simulink model "nncontroller_4_50"  (R2021a)
settings: Solver=VariableStepAuto  StartTime=0.0  StopTime=10.0  RelTol=1e-3
libraries: neural x206
(part 11 of 11)

== system nncontroller_4_50/Feed-Forward Neural Network/Layer 5/Delays 1 ==
  "p{5}" : Inport  PortDimensions=50
      mask Display: e = 0.06;c1 = [120 230 180]/255;c2 = ([120 230 180]+0)/(256+128);c3 = ([120 230 180]+128)/(256+128);patch([0 1 1 0],[0 0 1 1],c1);patch([0 1 1 1-e 1-e 0+e],[0 0 1 1-e 0+e 0+e],c2);patch([0 0 1 1-e 0+e 0+e],[0 1 1 1-e 1-e 0+e],c3);plot([0 1 1 0 0],[0 0 1 1 0]);
  mux : Mux  Inputs=1
      mask Display: e = 0.06;c1 = [120 150 230]/255;c2 = ([120 150 230]+0)/383;c3 = ([120 150 230]+128)/383;patch([0 1 1 0],[0 0 1 1],c1);patch([0 1 1 1-e 1-e 0+e],[0 0 1 1-e 0+e 0+e],c2);patch([0 0 1 1-e 0+e 0+e],[0 1 1 1-e 1-e 0+e],c3);plot([0 1 1 0 0],[0 0 1 1 0]);disp('Mux')
  "pd{5,4}" : Outport
      mask Display: e = 0.06;c1 = [120 230 180]/255;c2 = ([120 230 180]+0)/(256+128);c3 = ([120 230 180]+128)/(256+128);patch([0 1 1 0],[0 0 1 1],c1);patch([0 1 1 1-e 1-e 0+e],[0 0 1 1-e 0+e 0+e],c2);patch([0 0 1 1-e 0+e 0+e],[0 1 1 1-e 1-e 0+e],c3);plot([0 1 1 0 0],[0 0 1 1 0]);
  wires:
  "p{5}"/1 -> mux/1
  mux/1 -> "pd{5,4}"/1

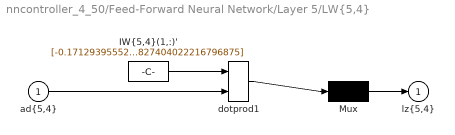
== system nncontroller_4_50/Feed-Forward Neural Network/Layer 5/LW{5,4} ==
  "ad{5,4}" : Inport  PortDimensions=50
      mask Display: e = 0.06;c1 = [120 230 180]/255;c2 = ([120 230 180]+0)/(256+128);c3 = ([120 230 180]+128)/(256+128);patch([0 1 1 0],[0 0 1 1],c1);patch([0 1 1 1-e 1-e 0+e],[0 0 1 1-e 0+e 0+e],c2);patch([0 0 1 1-e 0+e 0+e],[0 1 1 1-e 1-e 0+e],c3);plot([0 1 1 0 0],[0 0 1 1 0]);
  "IW{5,4}(1,:)'" : Constant  Value=[-0.1712939555266810298661539491149596869945526123046875;-0.72795551344690689887784174061380326747894287109375;0.406597786086664469973328550622682087123394012451171875;-0.86752023690311264036978400326916016638278961181640625;0.291551184054806622469868671032600104808807373046875;-0.7823842035386003868069337841006927192211151123046875;-0.9459670471661578705635520236683078110218048095703125;-0.301887099511520984318480032015941105782985687255859375;-0.362312844090777519401314066271879710257053375244140625;0.5028199275581730631756727234460413455963134765625;-0.87837751962319521314981329851434566080570220947265625;-0.289926976234542388421999703496112488210201263427734375;-0.7762515105937903836519353717449121177196502685546875;0.59758198869694301169630534786847420036792755126953125;0.6094541268886020102257816688506864011287689208984375;0.99514085054177059408431205156375654041767120361328125;-0.72455451572289220063538550675730220973491668701171875;-0.37830375588080566995330400459351949393749237060546875;-0.2354275486435387920725048616077401675283908843994140625;1.0042205230011191918748636453528888523578643798828125;0.69321866747018134891078489090432412922382354736328125;0.46433784951853152023204529541544616222381591796875;0.93726104060380410754049762545037083327770233154296875;0.252906313474891952797207750336383469402790069580078125;0.39013454713458373124268518949975259602069854736328125;0.76080914399647803225690267936442978680133819580078125;0.46840297437907174593618719882215373218059539794921875;0.92976033604283403466439494877704419195652008056640625;0.58910450754260512695736906607635319232940673828125;0.68743866930802643988585032275295816361904144287109375;0.6246040323366364166446373928920365869998931884765625;-0.4288077252260380500814562765299342572689056396484375;-0.4498523186398390993900875400868244469165802001953125;0.798384264007580668476293794810771942138671875;-0.52738475166148013340006173166329972445964813232421875;0.5197591612342986611139394881320185959339141845703125;0.5958154082946760521366513785324059426784515380859375;-0.8041283585005636336262568875099532306194305419921875;0.222925136027782855308032594621181488037109375;-0.6354100583953281589089101544232107698917388916015625;0.68212298596185216847942456297460012137889862060546875;-0.58446137624875127425383425361360423266887664794921875;-0.0962655766841698234959068258831393904983997344970703125;0.8598973975711088346685073702246882021427154541015625;0.316092898652422127359074011110351420938968658447265625;-0.2764815078060502973045231556170620024204254150390625;-0.67419866233348157980032056002528406679630279541015625;-0.6040478259355637202787647765944711863994598388671875;-0.8170124173290191915697278091101907193660736083984375;-0.46992077810438803719961242677527479827404022216796875]
      mask Display: e = 0.06;c1 = [120 150 230]/255;c2 = ([120 150 230]+0)/383;c3 = ([120 150 230]+128)/383;patch([0 1 1 0],[0 0 1 1],c1);patch([0 1 1 1-e 1-e 0+e],[0 0 1 1-e 0+e 0+e],c2);patch([0 0 1 1-e 0+e 0+e],[0 1 1 1-e 1-e 0+e],c3);plot([0 1 1 0 0],[0 0 1 1 0]);disp('weights');
  Mux : Mux  Inputs=1
      mask Display: e = 0.06;c1 = [120 150 230]/255;c2 = ([120 150 230]+0)/383;c3 = ([120 150 230]+128)/383;patch([0 1 1 0],[0 0 1 1],c1);patch([0 1 1 1-e 1-e 0+e],[0 0 1 1-e 0+e 0+e],c2);patch([0 0 1 1-e 0+e 0+e],[0 1 1 1-e 1-e 0+e],c3);plot([0 1 1 0 0],[0 0 1 1 0]);disp('Mux');
  dotprod1 : neural/Weight Functions/dotprod
  "lz{5,4}" : Outport
      mask Display: e = 0.06;c1 = [120 230 180]/255;c2 = ([120 230 180]+0)/(256+128);c3 = ([120 230 180]+128)/(256+128);patch([0 1 1 0],[0 0 1 1],c1);patch([0 1 1 1-e 1-e 0+e],[0 0 1 1-e 0+e 0+e],c2);patch([0 0 1 1-e 0+e 0+e],[0 1 1 1-e 1-e 0+e],c3);plot([0 1 1 0 0],[0 0 1 1 0]);
  wires:
  "IW{5,4}(1,:)'"/1 -> dotprod1/1
  "ad{5,4}"/1 -> dotprod1/2
  dotprod1/1 -> Mux/1
  Mux/1 -> "lz{5,4}"/1
